simulink model "uLaren"  (R2016a)
settings: Solver=FixedStepAuto  SolverMode=SingleTasking  StartTime=0.0  StopTime=inf  FixedStep=0.02  RelTol=1e-3
StartFcn:
  | setupPi
settings Model: Creator=idontknow  LastModifiedBy=idontknow
settings SolverCC: PositivePriorityOrder=on
settings OptimizationCC: OptimizeModelRefInitCode=on  MaxStackSize=64
settings DebuggingCC: ParameterTunabilityLossMsg=error  SFUnexpectedBacktrackingDiag=error  SFNoUnconditionalDefaultTransitionDiag=error
settings HardwareCC: ProdBitPerPointer=32  ProdLargestAtomicInteger=Long  ProdLargestAtomicFloat=Double  ProdWordSize=32  ProdHWDeviceType=ARM Compatible->ARM Cortex
settings RTWCC: SystemTargetFile=ert.tlc  HardwareBoard=Raspberry Pi  TLCOptions="-aInlineSetEventsForThisBaseRateFcn=TLC_FALSE -aSuppressMultiTaskScheduler=TLC_FALSE  -aRateBasedStepFcn=0"  TemplateMakefile=ert_default_tmf  GenerateReport=on  Toolchain=GNU GCC Raspberry Pi  IncludeHyperlinkInReport=on  LaunchReport=on  GenerateTraceInfo=on  GenerateTraceReport=on  GenerateTraceReportSl=on  GenerateTraceReportSf=on  GenerateTraceReportEml=on
settings CodeAppCC: ForceParamTrailComments=on  IgnoreCustomStorageClasses=off  OperatorAnnotations=on  SimulinkDataObjDesc=on  SFDataObjDesc=on  MATLABFcnDesc=on  InsertBlockDesc=on  MATLABSourceComments=on
settings ERTTargetCC: SupportVariableSizeSignals=on
settings ConfigComp: CovMetricSettings=dwe  CovHtmlReporting=off  CovSaveCumulativeToWorkspaceVar=off  CovSaveSingleToWorkspaceVar=off  CovExternalEMLEnable=on

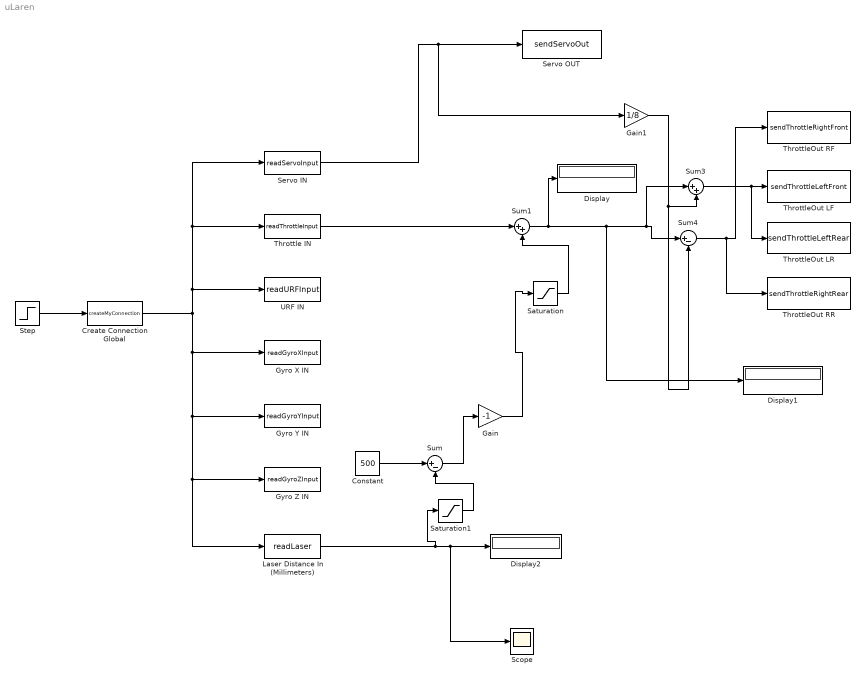
== system uLaren ==
  Constant : Constant  Value=500
  Create Connection Global : MATLABFcn  MATLABFcn=createMyConnection
  Display : Display
  Display1 : Display
  Display2 : Display
  Gain : Gain  Gain=-1
  Gain1 : Gain  Gain=1/8
  Gyro X IN : MATLABFcn  MATLABFcn=readGyroXInput
  Gyro Y IN : MATLABFcn  MATLABFcn=readGyroYInput
  Gyro Z IN : MATLABFcn  MATLABFcn=readGyroZInput
  Laser Distance In (Millimeters) : MATLABFcn  MATLABFcn=readLaser
  Saturation : Saturate  UpperLimit=100  LowerLimit=-500
  Saturation1 : Saturate  UpperLimit=500  LowerLimit=0
  Scope : Scope
  "Servo IN " : MATLABFcn  MATLABFcn=readServoInput  OutputSignalType=real
  Servo OUT : MATLABFcn  MATLABFcn=sendServoOut  OutputDimensions=0
  Step : Step  SampleTime=.02
  Sum : Sum  Inputs=|+-
  Sum1 : Sum  Inputs=|++
  Sum3 : Sum  Inputs=|++
  Sum4 : Sum  Inputs=|+-
  Throttle IN : MATLABFcn  MATLABFcn=readThrottleInput
  ThrottleOut LF : MATLABFcn  MATLABFcn=sendThrottleLeftFront  OutputDimensions=0
  ThrottleOut LR : MATLABFcn  MATLABFcn=sendThrottleLeftRear  OutputDimensions=0
  ThrottleOut RF : MATLABFcn  MATLABFcn=sendThrottleRightFront  OutputDimensions=0
  ThrottleOut RR : MATLABFcn  MATLABFcn=sendThrottleRightRear  OutputDimensions=0
  URF IN : MATLABFcn  MATLABFcn=readURFInput
  wires:
  Step/1 -> Create Connection Global/1
  Create Connection Global/1 -> Laser Distance In (Millimeters)/1, Gyro Z IN/1, Gyro Y IN/1, Gyro X IN/1, URF IN/1, Throttle IN/1, "Servo IN "/1
  "Servo IN "/1 -> Gain1/1, Servo OUT/1
  Laser Distance In (Millimeters)/1 -> Scope/1, Display2/1, Saturation1/1
  Constant/1 -> Sum/1
  Sum/1 -> Gain/1
  Gain/1 -> Saturation/1
  Throttle IN/1 -> Sum1/1
  Saturation/1 -> Sum1/2
  Saturation1/1 -> Sum/2
  Sum1/1 -> Display/1, Display1/1, Sum3/1, Sum4/1
  Gain1/1 -> Sum4/2, Sum3/2
  Sum4/1 -> ThrottleOut RR/1, ThrottleOut RF/1
  Sum3/1 -> ThrottleOut LF/1, ThrottleOut LR/1
